simulink model "DigitalTwinUAV_R22"  (R2022a)
settings: Solver=VariableStepAuto  StartTime=0.0  StopTime=90  FixedStep=0.01  RelTol=1e-3
PreLoadFcn:
  | addpath(genpath('./images'));
InitFcn:
  | addpath(genpath('./model'));
  | QuadcopterParameters;
values from neighbouring files (symbols this model uses):
  m = 1.5    [QuadcopterParameters.m]    (also in QuadcopterParameters1.m; QuadcopterParameters_Gen.m = 1.2)
  trajColor = [0 0 0;              1 0 0;              0 0 1;]    [QuadcopterParameters.m]    (also in QuadcopterParameters1.m; QuadcopterParameters_Gen.m)
  xrot = 0    [QuadcopterParameters.m]    (also in QuadcopterParameters1.m; QuadcopterParameters_Gen.m)
  yrot = 0    [QuadcopterParameters.m]    (also in QuadcopterParameters1.m; QuadcopterParameters_Gen.m)
  zrot = 0    [QuadcopterParameters.m]    (also in QuadcopterParameters1.m; QuadcopterParameters_Gen.m)
undefined symbols (not defined in the file or in its folder): crane, excavator, uav, X, Y, Z
libraries: sm_lib x23, nesl_utility x1
(part 1 of 2)
settings Model: Creator=ADMIN  LastModifiedBy=ADMIN
settings SolverCC: MinimalZcImpactIntegration=on
settings SimscapeCC: SimscapeCompileComponentReuse=on
settings ExplorerConfigSet: InternalSimMechanicsExplorerSettings="<ExplorerConfiguration><canonicalview>default</canonicalview><AnimationSetting><BasePlaybackSpeed>1.0</BasePlaybackSpeed><PlaybackSpeedFactor>1.0</PlaybackSpeedFactor></AnimationSetting><TilePanel><TileInfo><Tiles Columns=\"1\" Count=\"1\" Rows=\"1\"><Column Weight=\"1\"/><Row Weight=\"1\"/><Tile Height=\"1\" Width=\"1\" X=\"0\" Y=\"0\"/></Tiles></TileInfo><SceneInfo><SceneViewer><BGColor><R>0.27843138575553894</R><G>0.756862759590148926</G><B>1</B></BGColor><Camera><DoPerspective>on</DoPerspective><Position><X>138.89503174773705</X><Y>141.338904454019598</Y><Z>58.1618377405307001</Z></Position><Center><X>60.3194201572761557</X><Y>73.694454858331909</Y><Z>-0.0339667202272622148</Z></Center><Up><X>-0.356422741563376222</X><Y>-0.336016505355418327</Y><Z>0.871811755727794013</Z></Up><ViewLimDist>1</ViewLimDist><YLim>0.466307658154998583</YLim><XLim>0.993847635057623302</XLim></Camera></SceneViewer></SceneInfo></TilePanel><MechEditorPanel><Cameras><Camera><Id>Camera1</Id><Value><Name>Camera</Name><NativeCamera><PositionKeyframeSet><Keyframe><Time>0</Time><Value><X>427.15819708198001</X><Y>-427.15819423097219</Y><Z>426.90819247014201</Z></Value></Keyframe><Keyframe><Time>0.79457934452222712</Time><Value><X>390.94235477737851</X><Y>-386.70665235425116</Y><Z>390.0308137752491</Z></Value></Keyframe><Keyframe><Time>2.7607911592394796</Time><Value><X>158.64332905928893</X><Y>-123.54772038663614</Y><Z>149.97829764303876</Z></Value></Keyframe><Keyframe><Time>5.5687271331598325</Time><Value><X>18.352849951551754</X><Y>24.396360824115767</Y><Z>18.562507619437909</Z></Value></Keyframe><Keyframe><Time>8.621944778587002</Time><Value><X>20.826011553668287</X><Y>30.414284305635885</Y><Z>22.10726949884149</Z></Value></Keyframe><Keyframe><Time>21.446938827871989</Time><Value><X>19.889419356045895</X><Y>44.10598770409257</Y><Z>15.738331202819449</Z></Value></Keyframe><Keyframe><Time>27.401526741577165</Time><Value><X>21.930325513031203</X><Y>49.554645689571032</Y><Z>15.972170552776927</Z></Value></Keyframe><Keyframe><Time>34.605538577791457</Time><Value><X>26.025912835327635</X><Y>57.985685802266083</Y><Z>15.892067554830771</Z></Value></Keyframe><Keyframe><Time>45.499317901054738</Time><Value><X>31.896560076715794</X><Y>65.244002145148229</Y><Z>15.465340540520041</Z></Value></Keyframe><Keyframe><Time>55.071901613661723</Time><Value><X>37.240526947587739</X><Y>68.058216295740905</Y><Z>16.878264808436938</Z></Value></Keyframe><Keyframe><Time>62.860219848906418</Time><Value><X>35.065406183068731</X><Y>62.163143721032611</Y><Z>16.14648566291422</Z></Value></Keyframe><Keyframe><Time>70.548436312612282</Time><Value><X>41.431101082419787</X><Y>65.763582084873633</Y><Z>15.666397795239471</Z></Value></Keyframe><Keyframe><Time>78.126717813603349</Time><Value><X>42.555026223671902</X><Y>67.92319371264098</Y><Z>16.748697346533454</Z></Value></Keyframe><Keyframe><Time>84.304620203487019</Time><Value><X>47.88954698511801</X><Y>72.641324967288227</Y><Z>16.299206866506246</Z></Value></Keyframe><Keyframe><Time>89.667208950866709</Time><Value><X>63.197259172121463</X><Y>84.566139055302173</Y><Z>18.486390887992304</Z></Value></Keyframe><Keyframe><Time>92.959131386818399</Time><Value><X>69.956308832017754</X><Y>89.839406171374179</Y><Z>19.43507026407455</Z></Value></Keyframe><Keyframe><Time>97.322347567853896</Time><Value><X>69.956308832017754</X><Y>89.839406171374179</Y><Z>19.43507026407455</Z></Value></Keyframe><Keyframe><Time>98.712529870538134</Time><Value><X>74.584383228853454</X><Y>87.281767315743537</Y><Z>18.165708290173569</Z></Value></Keyframe><Keyframe><Time>99.998699176458231</Time><Value><X>91.399732222435318</X><Y>137.62730154690249</Y><Z>39.166257857095417</Z></Value></Keyframe></PositionKeyframeSet><CenterKeyframeSet><Keyframe><Time>0</Time><Value><X>0.083335820948605033</X><Y>-0.083332969940784096</Y><Z>-0.16666879088938913</Z></Value></Keyframe><Keyframe><Time>0.79457934452222712</Time><Value><X>0.57379571983329924</X><Y>3.6619067032940507</Y><Z>-0.33774528229611178</Z></Value></Keyframe><Keyframe><Time>2.7607911592394796</Time><Value><X>8.66462376881978</X><Y>26.430984903833007</Y><Z>-0.00040764743039289897</Z></Value></Keyframe><Keyframe><Time>5.5687271331598325</Time><Value><X>-0.20970812157613494</X><Y>42.958918897243649</Y><Z>-5.0453689972584925e-05</Z></Value></Keyframe><Keyframe><Time>8.621944778587002</Time><Value><X>-1.2813180336776462</X><Y>52.521613892981804</Y><Z>-6.0088504437061374e-05</Z></Value></Keyframe><Keyframe><Time>21.446938827871989</Time><Value><X>4.1510453757688168</X><Y>59.844361684369609</Y><Z>-4.2777457625930992e-05</Z></Value></Keyframe><Keyframe><Time>27.401526741577165</Time><Value><X>5.958111547211292</X><Y>65.526859655390879</Y><Z>-4.3413042980944283e-05</Z></Value></Keyframe><Keyframe><Time>34.605538577791457</Time><Value><X>10.133802085177258</X><Y>73.877796552416413</Y><Z>-4.3195319602062909e-05</Z></Value></Keyframe><Keyframe><Time>45.499317901054738</Time><Value><X>31.445175359024709</X><Y>65.695386862839314</Y><Z>15.013955822828954</Z></Value></Keyframe><Keyframe><Time>55.071901613661723</Time><Value><X>57.580363961468976</X><Y>79.121527581700704</Y><Z>-4.337800287146365e-05</Z></Value></Keyframe><Keyframe><Time>62.860219848906418</Time><Value><X>56.144668811679956</X><Y>45.463359961310942</Y><Z>-6.1925334591705905e-05</Z></Value></Keyframe><Keyframe><Time>70.548436312612282</Time><Value><X>70.673607091545776</X><Y>33.834095876567901</Y><Z>-0.00016262240450970467</Z></Value></Keyframe><Keyframe><Time>78.126717813603349</Time><Value><X>73.053878820458976</X><Y>31.844243209726066</Y><Z>-0.00018157159788501076</Z></Value></Keyframe><Keyframe><Time>84.304620203487019</Time><Value><X>77.569891514658522</X><Y>37.530637514621176</Y><Z>-0.00017669869923864212</Z></Value></Keyframe><Keyframe><Time>89.667208950866709</Time><Value><X>96.860397210505056</X><Y>44.743962558486032</Y><Z>-0.00020040982668589891</Z></Value></Keyframe><Keyframe><Time>92.959131386818399</Time><Value><X>105.34696226184363</X><Y>47.97364649046682</Y><Z>-0.00021069440148835383</Z></Value></Keyframe><Keyframe><Time>97.322347567853896</Time><Value><X>105.34696226184349</X><Y>47.973646490466983</Y><Z>-0.00021069440141019413</Z></Value></Keyframe><Keyframe><Time>98.712529870538134</Time><Value><X>74.078241101652537</X><Y>85.981985203045838</Y><Z>17.6855975838644</Z></Value></Keyframe><Keyframe><Time>99.998699176458231</Time><Value><X>68.472813135391121</X><Y>78.75055976409854</Y><Z>17.418494284741232</Z></Value></Keyframe></CenterKeyframeSet><UpVectorKeyframeSet><Keyframe><Time>0</Time><Value><X>-0.40824829046386302</X><Y>0.40824829046386302</Y><Z>0.81649658092772603</Z></Value></Keyframe><Keyframe><Time>0.79457934452222712</Time><Value><X>-0.40824829046386302</X><Y>0.40824829046386302</Y><Z>0.81649658092772603</Z></Value></Keyframe><Keyframe><Time>2.7607911592394796</Time><Value><X>-0.40824829046386307</X><Y>0.40824829046386307</Y><Z>0.81649658092772615</Z></Value></Keyframe><Keyframe><Time>5.5687271331598325</Time><Value><X>-0.40824829046386302</X><Y>0.40824829046386302</Y><Z>0.81649658092772626</Z></Value></Keyframe><Keyframe><Time>8.621944778587002</Time><Value><X>-0.40824829046386302</X><Y>0.40824829046386302</Y><Z>0.81649658092772603</Z></Value></Keyframe><Keyframe><Time>21.446938827871989</Time><Value><X>-0.40824829046386329</X><Y>0.40824829046386335</Y><Z>0.81649658092772581</Z></Value></Keyframe><Keyframe><Time>27.401526741577165</Time><Value><X>-0.40824829046386346</X><Y>0.40824829046386346</Y><Z>0.81649658092772548</Z></Value></Keyframe><Keyframe><Time>34.605538577791457</Time><Value><X>-0.40824829046386324</X><Y>0.40824829046386335</Y><Z>0.81649658092772559</Z></Value></Keyframe><Keyframe><Time>45.499317901054738</Time><Value><X>-0.40824829046386291</X><Y>0.40824829046386307</Y><Z>0.81649658092772603</Z></Value></Keyframe><Keyframe><Time>55.071901613661723</Time><Value><X>0.54474303700342208</X><Y>0.22917420964799837</Y><Z>0.80668098110002795</Z></Value></Keyframe><Keyframe><Time>62.860219848906418</Time><Value><X>0.33216731732567528</X><Y>-0.40455279321782145</Y><Z>0.85205745745244355</Z></Value></Keyframe><Keyframe><Time>70.548436312612282</Time><Value><X>0.22596689908931417</X><Y>-0.2544284640580029</Y><Z>0.94032181575939477</Z></Value></Keyframe><Keyframe><Time>78.126717813603349</Time><Value><X>0.24849257206902248</X><Y>-0.22707675815979272</Y><Z>0.94164090158093749</Z></Value></Keyframe><Keyframe><Time>84.304620203487019</Time><Value><X>0.24849257206902248</X><Y>-0.22707675815979275</Y><Z>0.94164090158093749</Z></Value></Keyframe><Keyframe><Time>89.667208950866709</Time><Value><X>0.24849257206902245</X><Y>-0.22707675815979272</Y><Z>0.94164090158093749</Z></Value></Keyframe><Keyframe><Time>92.959131386818399</Time><Value><X>0.24849257206902245</X><Y>-0.22707675815979272</Y><Z>0.94164090158093749</Z></Value></Keyframe><Keyframe><Time>97.322347567853896</Time><Value><X>0.24849257206902245</X><Y>-0.2270767581597927</Y><Z>0.94164090158093749</Z></Value></Keyframe><Keyframe><Time>98.712529870538134</Time><Value><X>-0.11527700489361359</X><Y>-0.30437604885319575</Y><Z>0.945550862210635</Z></Value></Keyframe><Keyframe><Time>99.998699176458231</Time><Value><X>-0.11527700489361427</X><Y>-0.30437604885319752</Y><Z>0.94555086221063411</Z></Value></Keyframe></UpVectorKeyframeSet></NativeCamera></Value></Camera><Camera><Id>Camera2</Id><Value><Name>Camera2</Name><NativeCamera><PositionKeyframeSet><Keyframe><Time>0</Time><Value><X>229.42211701613911</X><Y>-181.57056116872968</Y><Z>204.32036374857904</Z></Value></Keyframe><Keyframe><Time>1.000273018622585</Time><Value><X>197.55127895537666</X><Y>-148.90451616468175</Y><Z>172.77519677524185</Z></Value></Keyframe><Keyframe><Time>1.9998413608981176</Time><Value><X>152.00964089221299</X><Y>-103.76251203481223</Y><Z>129.85617953038943</Z></Value></Keyframe><Keyframe><Time>2.9997698665509209</Time><Value><X>91.305579739639839</X><Y>-43.282088723920879</Y><Z>76.593292484691659</Z></Value></Keyframe><Keyframe><Time>4.0000437696161804</Time><Value><X>63.675921698844178</X><Y>-16.182993482292915</Y><Z>53.58702589586548</Z></Value></Keyframe><Keyframe><Time>5.0001784288957127</Time><Value><X>30.124862570999188</X><Y>14.013191865709302</Y><Z>25.811716641985729</Z></Value></Keyframe><Keyframe><Time>6.0001514418482849</Time><Value><X>23.245853605889877</X><Y>21.271258776668272</Y><Z>19.318526585402044</Z></Value></Keyframe><Keyframe><Time>7.0000336661717562</Time><Value><X>26.868198636186534</X><Y>25.847341414168035</Y><Z>20.272264192605149</Z></Value></Keyframe><Keyframe><Time>8.000135993662056</Time><Value><X>26.868198636186534</X><Y>25.847341414168035</Y><Z>20.272264192605149</Z></Value></Keyframe><Keyframe><Time>12.000060521855515</Time><Value><X>26.327006126208872</X><Y>27.710686973014656</Y><Z>22.676802261429437</Z></Value></Keyframe><Keyframe><Time>14.999735667122877</Time><Value><X>28.295728944359858</X><Y>27.480602511595009</Y><Z>20.477994981858799</Z></Value></Keyframe><Keyframe><Time>16.000205697859094</Time><Value><X>30.310341141247953</X><Y>29.879687394354729</Y><Z>20.862467667730424</Z></Value></Keyframe><Keyframe><Time>18</Time><Value><X>26.770305336655007</X><Y>35.477008620321833</Y><Z>18.099995586746186</Z></Value></Keyframe><Keyframe><Time>20.00000304433263</Time><Value><X>27.472962547810489</X><Y>37.810046819920885</Y><Z>19.730376575189759</Z></Value></Keyframe><Keyframe><Time>22.000224197946089</Time><Value><X>26.9792421697192</X><Y>37.813168521453861</Y><Z>19.792629719475226</Z></Value></Keyframe><Keyframe><Time>24.00016511781271</Time><Value><X>24.889252072130148</X><Y>35.375391905924594</Y><Z>19.531772772823498</Z></Value></Keyframe><Keyframe><Time>26.000093825701278</Time><Value><X>23.428642671004315</X><Y>37.197471869241348</Y><Z>17.738764614919702</Z></Value></Keyframe><Keyframe><Time>27.999962847707238</Time><Value><X>20.387005350891794</X><Y>42.79597426548974</Y><Z>16.352519575890927</Z></Value></Keyframe><Keyframe><Time>29.999690502428876</Time><Value><X>19.277686757978806</X><Y>43.962422440853544</Y><Z>16.146129384446127</Z></Value></Keyframe><Keyframe><Time>31.999734624362802</Time><Value><X>19.72713372758853</X><Y>48.573829120962806</Y><Z>18.193453440233878</Z></Value></Keyframe><Keyframe><Time>33.999673255119724</Time><Value><X>19.782458532238007</X><Y>52.112301987038968</Y><Z>19.642549513946232</Z></Value></Keyframe><Keyframe><Time>36</Time><Value><X>21.55325105949694</X><Y>53.949829712966483</Y><Z>19.171654687490552</Z></Value></Keyframe><Keyframe><Time>37.99983496478324</Time><Value><X>23.437474942885132</X><Y>55.627893150481249</Y><Z>16.994152381120042</Z></Value></Keyframe><Keyframe><Time>39.999704023181188</Time><Value><X>24.998911581156065</X><Y>62.488557443752292</Y><Z>18.940639854790781</Z></Value></Keyframe><Keyframe><Time>42.000166465258886</Time><Value><X>28.409434539739252</X><Y>69.214963954081696</Y><Z>20.058059863527468</Z></Value></Keyframe><Keyframe><Time>43.999717964839682</Time><Value><X>34.699289096189688</X><Y>70.961283734018451</Y><Z>18.466447327852634</Z></Value></Keyframe><Keyframe><Time>45.999916464499805</Time><Value><X>36.40543007932564</X><Y>71.857960605414263</Y><Z>17.64562444618441</Z></Value></Keyframe><Keyframe><Time>48.000128581837849</Time><Value><X>39.43057749066287</X><Y>72.257422850905826</Y><Z>18.739347841870078</Z></Value></Keyframe><Keyframe><Time>49.99992478618293</Time><Value><X>43.422403550355781</X><Y>73.212796107446692</Y><Z>16.439241194456741</Z></Value></Keyframe><Keyframe><Time>51.999674329862636</Time><Value><X>46.934269420811198</X><Y>73.396555233271229</Y><Z>16.005507762443312</Z></Value></Keyframe><Keyframe><Time>54</Time><Value><X>49.102122803066699</X><Y>78.463229181998017</Y><Z>17.60108062581412</Z></Value></Keyframe><Keyframe><Time>56.000405512171703</Time><Value><X>50.933014881578096</X><Y>78.223728424998271</Y><Z>17.735828542058144</Z></Value></Keyframe><Keyframe><Time>57.999833678854806</Time><Value><X>53.835348032966493</X><Y>76.818838883930439</Y><Z>16.905995306639007</Z></Value></Keyframe><Keyframe><Time>59.99979126155737</Time><Value><X>61.626438596615735</X><Y>77.152448025005825</Y><Z>20.076073882268343</Z></Value></Keyframe><Keyframe><Time>61.999963873580292</Time><Value><X>61.969626521341368</X><Y>78.283733041699435</Y><Z>18.229640876326858</Z></Value></Keyframe><Keyframe><Time>65.999733038800883</Time><Value><X>69.166882183227898</X><Y>88.998353875388489</Y><Z>24.848351588577749</Z></Value></Keyframe><Keyframe><Time>70.000024012162029</Time><Value><X>72.56719371536758</X><Y>87.651305544240998</Y><Z>21.960175902186091</Z></Value></Keyframe><Keyframe><Time>75.000250424912963</Time><Value><X>80.058475334563909</X><Y>92.123433446463935</Y><Z>23.018878398528422</Z></Value></Keyframe><Keyframe><Time>80.000129153530565</Time><Value><X>81.377418765025041</X><Y>91.152346896609615</Y><Z>22.449006776150824</Z></Value></Keyframe><Keyframe><Time>85.00016728403746</Time><Value><X>83.985608228435296</X><Y>87.819241830809133</Y><Z>23.05563029704135</Z></Value></Keyframe><Keyframe><Time>86.000313905552019</Time><Value><X>94.607344859457129</X><Y>98.816411737799271</Y><Z>29.324817264882864</Z></Value></Keyframe><Keyframe><Time>87.000040311365154</Time><Value><X>107.47852215936517</X><Y>110.35675145021976</Y><Z>36.94655917351227</Z></Value></Keyframe><Keyframe><Time>88.000098835330618</Time><Value><X>117.80884802291686</X><Y>118.56459591723726</Y><Z>41.509985959976191</Z></Value></Keyframe><Keyframe><Time>89.000164588923155</Time><Value><X>138.89503174773705</X><Y>141.3389044540196</Y><Z>58.1618377405307</Z></Value></Keyframe><Keyframe><Time>90</Time><Value><X>138.89503174773705</X><Y>141.3389044540196</Y><Z>58.1618377405307</Z></Value></Keyframe></PositionKeyframeSet><CenterKeyframeSet><Keyframe><Time>0</Time><Value><X>31.551215256709213</X><Y>16.300340590700216</Y><Z>6.4494619891492846</Z></Value></Keyframe><Keyframe><Time>1.000273018622585</Time><Value><X>31.225629910397572</X><Y>17.421132880297336</Y><Z>6.449547730262907</Z></Value></Keyframe><Keyframe><Time>1.9998413608981176</Time><Value><X>28.603125747811816</X><Y>19.644003109588937</Y><Z>6.4496643859883562</Z></Value></Keyframe><Keyframe><Time>2.9997698665509209</Time><Value><X>21.162096411742439</X><Y>26.861394603976521</Y><Z>6.4498091567943305</Z></Value></Keyframe><Keyframe><Time>4.0000437696161804</Time><Value><X>10.097994763739074</X><Y>37.39493345281219</Y><Z>0.0090989607604328171</Z></Value></Keyframe><Keyframe><Time>5.0001784288957127</Time><Value><X>4.2543460249819205</X><Y>39.883708411726559</Y><Z>-0.05879990403151325</Z></Value></Keyframe><Keyframe><Time>6.0001514418482849</Time><Value><X>3.8660014095456816</X><Y>40.651110973012464</Y><Z>-0.061325610942130737</Z></Value></Keyframe><Keyframe><Time>7.0000336661717562</Time><Value><X>8.6220160008767692</X><Y>44.0935240494778</Y><Z>2.0260815572954023</Z></Value></Keyframe><Keyframe><Time>8.000135993662056</Time><Value><X>8.6220160008767692</X><Y>44.0935240494778</Y><Z>2.0260815572954023</Z></Value></Keyframe><Keyframe><Time>12.000060521855515</Time><Value><X>3.6196002136333156</X><Y>50.418092885590212</Y><Z>-0.03060365114610164</Z></Value></Keyframe><Keyframe><Time>14.999735667122877</Time><Value><X>9.8435740796902387</X><Y>45.932757376264625</Y><Z>2.025840117189194</Z></Value></Keyframe><Keyframe><Time>16.000205697859094</Time><Value><X>9.3757361975952556</X><Y>50.814292338007419</Y><Z>-0.072137275922251831</Z></Value></Keyframe><Keyframe><Time>18</Time><Value><X>8.5950745814058997</X><Y>53.652239375570929</Y><Z>-0.075235168502903349</Z></Value></Keyframe><Keyframe><Time>20.00000304433263</Time><Value><X>7.6933622646033051</X><Y>57.589647103128058</Y><Z>-0.049223708017400725</Z></Value></Keyframe><Keyframe><Time>22.000224197946089</Time><Value><X>7.782901084608234</X><Y>63.428094772265339</Y><Z>-0.038654727826529012</Z></Value></Keyframe><Keyframe><Time>24.00016511781271</Time><Value><X>13.913441370701982</X><Y>66.048311344047619</Y><Z>-0.092996799423143983</Z></Value></Keyframe><Keyframe><Time>26.000093825701278</Time><Value><X>23.072997760502972</X><Y>76.610494481889674</Y><Z>-0.14044226985273767</Z></Value></Keyframe><Keyframe><Time>27.999962847707238</Time><Value><X>46.056529688525444</X><Y>98.918869182276225</Y><Z>-0.14817845045401867</Z></Value></Keyframe><Keyframe><Time>29.999690502428876</Time><Value><X>38.716876529679176</X><Y>72.170423114431159</Y><Z>2.6247209653232257</Z></Value></Keyframe><Keyframe><Time>31.999734624362802</Time><Value><X>45.151887248357326</X><Y>74.962821820866424</Y><Z>-0.14866172727078464</Z></Value></Keyframe><Keyframe><Time>33.999673255119724</Time><Value><X>43.931163511354093</X><Y>67.582519550125397</Y><Z>-0.12866311492846805</Z></Value></Keyframe><Keyframe><Time>36</Time><Value><X>43.067358977399621</X><Y>65.689847250674404</Y><Z>-0.14765266506854857</Z></Value></Keyframe><Keyframe><Time>37.99983496478324</Time><Value><X>49.609993385732579</X><Y>60.617525110879157</Y><Z>-0.17407851231168436</Z></Value></Keyframe><Keyframe><Time>39.999704023181188</Time><Value><X>51.174089651313913</X><Y>54.359329955310301</Y><Z>-0.13671416647383694</Z></Value></Keyframe><Keyframe><Time>42.000166465258886</Time><Value><X>50.696412624780663</X><Y>51.690721304467345</Y><Z>-0.19360313930595296</Z></Value></Keyframe><Keyframe><Time>43.999717964839682</Time><Value><X>48.011280497921405</X><Y>51.102412583964153</Y><Z>-0.16139757887929562</Z></Value></Keyframe><Keyframe><Time>45.999916464499805</Time><Value><X>42.027850149919999</X><Y>46.970089378998651</Y><Z>-0.15914948743381885</Z></Value></Keyframe><Keyframe><Time>48.000128581837849</Time><Value><X>39.876142820446589</X><Y>48.019983028776402</Y><Z>0.23639313961458086</Z></Value></Keyframe><Keyframe><Time>49.99992478618293</Time><Value><X>43.155499075415847</X><Y>39.116884003467959</Y><Z>-0.16719766176567674</Z></Value></Keyframe><Keyframe><Time>51.999674329862636</Time><Value><X>46.674274865613164</X><Y>40.183356003321087</Y><Z>-0.17100514472535622</Z></Value></Keyframe><Keyframe><Time>54</Time><Value><X>40.19857623926984</X><Y>40.436259613424383</Y><Z>-0.17876690208317214</Z></Value></Keyframe><Keyframe><Time>56.000405512171703</Time><Value><X>30.565909477925825</X><Y>46.68510342886735</Y><Z>-0.10370858691696228</Z></Value></Keyframe><Keyframe><Time>57.999833678854806</Time><Value><X>34.360890580665838</X><Y>46.662486352800599</Y><Z>-0.1516719416811334</Z></Value></Keyframe><Keyframe><Time>59.99979126155737</Time><Value><X>34.620682256769918</X><Y>52.339801741754989</Y><Z>-0.14573991684069298</Z></Value></Keyframe><Keyframe><Time>61.999963873580292</Time><Value><X>37.429707408008767</X><Y>55.736675847070806</Y><Z>-0.14576282317352351</Z></Value></Keyframe><Keyframe><Time>65.999733038800883</Time><Value><X>35.747406970283912</X><Y>58.292840317630379</Y><Z>-0.17603197304744356</Z></Value></Keyframe><Keyframe><Time>70.000024012162029</Time><Value><X>42.962834940698002</X><Y>60.451086691843429</Y><Z>-0.20746210986618863</Z></Value></Keyframe><Keyframe><Time>75.000250424912963</Time><Value><X>49.082196705445583</X><Y>63.662706958248734</Y><Z>-0.17604829579010328</Z></Value></Keyframe><Keyframe><Time>80.000129153530565</Time><Value><X>51.181542102007761</X><Y>63.408646723078604</Y><Z>-0.16155771596307034</Z></Value></Keyframe><Keyframe><Time>85.00016728403746</Time><Value><X>52.961369683396633</X><Y>59.314450202757428</Y><Z>-0.17520861085703388</Z></Value></Keyframe><Keyframe><Time>86.000313905552019</Time><Value><X>55.165568234182842</X><Y>62.577661751672807</Y><Z>-0.20904406399046849</Z></Value></Keyframe><Keyframe><Time>87.000040311365154</Time><Value><X>58.034445661262353</X><Y>64.927978209780093</Y><Z>-0.076988540954268103</Z></Value></Keyframe><Keyframe><Time>88.000098835330618</Time><Value><X>62.185868062220734</X><Y>67.458701691688489</Y><Z>-0.14030257710807348</Z></Value></Keyframe><Keyframe><Time>89.000164588923155</Time><Value><X>60.319420157276156</X><Y>73.694454858331909</Y><Z>-0.033966720227262215</Z></Value></Keyframe><Keyframe><Time>90</Time><Value><X>60.319420157276156</X><Y>73.694454858331909</Y><Z>-0.033966720227262215</Z></Value></Keyframe></CenterKeyframeSet><UpVectorKeyframeSet><Keyframe><Time>0</Time><Value><X>-0.40824829046386285</X><Y>0.40824829046386285</Y><Z>0.81649658092772637</Z></Value></Keyframe><Keyframe><Time>1.000273018622585</Time><Value><X>-0.40824829046386285</X><Y>0.40824829046386285</Y><Z>0.81649658092772637</Z></Value></Keyframe><Keyframe><Time>1.9998413608981176</Time><Value><X>-0.4082482904638628</X><Y>0.4082482904638628</Y><Z>0.81649658092772615</Z></Value></Keyframe><Keyframe><Time>2.9997698665509209</Time><Value><X>-0.4082482904638628</X><Y>0.4082482904638628</Y><Z>0.81649658092772637</Z></Value></Keyframe><Keyframe><Time>4.0000437696161804</Time><Value><X>-0.4082482904638628</X><Y>0.4082482904638628</Y><Z>0.81649658092772637</Z></Value></Keyframe><Keyframe><Time>5.0001784288957127</Time><Value><X>-0.4082482904638628</X><Y>0.40824829046386285</Y><Z>0.81649658092772626</Z></Value></Keyframe><Keyframe><Time>6.0001514418482849</Time><Value><X>-0.40824829046386274</X><Y>0.4082482904638628</Y><Z>0.81649658092772626</Z></Value></Keyframe><Keyframe><Time>7.0000336661717562</Time><Value><X>-0.4082482904638628</X><Y>0.4082482904638628</Y><Z>0.81649658092772637</Z></Value></Keyframe><Keyframe><Time>8.000135993662056</Time><Value><X>-0.4082482904638628</X><Y>0.4082482904638628</Y><Z>0.81649658092772637</Z></Value></Keyframe><Keyframe><Time>12.000060521855515</Time><Value><X>-0.40824829046386285</X><Y>0.4082482904638628</Y><Z>0.81649658092772626</Z></Value></Keyframe><Keyframe><Time>14.999735667122877</Time><Value><X>-0.40824829046386285</X><Y>0.4082482904638628</Y><Z>0.81649658092772626</Z></Value></Keyframe><Keyframe><Time>16.000205697859094</Time><Value><X>-0.40824829046386285</X><Y>0.40824829046386274</Y><Z>0.81649658092772648</Z></Value></Keyframe><Keyframe><Time>18</Time><Value><X>-0.40824829046386291</X><Y>0.4082482904638628</Y><Z>0.81649658092772626</Z></Value></Keyframe><Keyframe><Time>20.00000304433263</Time><Value><X>-0.40824829046386285</X><Y>0.40824829046386274</Y><Z>0.81649658092772626</Z></Value></Keyframe><Keyframe><Time>22.000224197946089</Time><Value><X>-0.2076415760691887</X><Y>0.49678828253428997</Y><Z>0.8426662318048197</Z></Value></Keyframe><Keyframe><Time>24.00016511781271</Time><Value><X>-0.10349153115718084</X><Y>0.5095047257952674</Y><Z>0.85422153881240426</Z></Value></Keyframe><Keyframe><Time>26.000093825701278</Time><Value><X>0.01724342445728275</X><Y>0.41318482538090323</Y><Z>0.91048391769868098</Z></Value></Keyframe><Keyframe><Time>27.999962847707238</Time><Value><X>0.067872605599444649</X><Y>0.25272182893157097</Y><Z>0.96515542095075224</Z></Value></Keyframe><Keyframe><Time>29.999690502428876</Time><Value><X>0.1909138696933684</X><Y>0.31420726264793852</Y><Z>0.92996004777516816</Z></Value></Keyframe><Keyframe><Time>31.999734624362802</Time><Value><X>0.25943152749458853</X><Y>0.37007666749622292</Y><Z>0.89204178305543236</Z></Value></Keyframe><Keyframe><Time>33.999673255119724</Time><Value><X>0.46197420427831631</X><Y>0.33062684214562105</Y><Z>0.82296155793222292</Z></Value></Keyframe><Keyframe><Time>36</Time><Value><X>0.60437195743408978</X><Y>0.17243437041644957</Y><Z>0.77781805389587721</Z></Value></Keyframe><Keyframe><Time>37.99983496478324</Time><Value><X>0.53647232249382293</X><Y>0.07747352789652838</Y><Z>0.8403542703368323</Z></Value></Keyframe><Keyframe><Time>39.999704023181188</Time><Value><X>0.53033272477981597</X><Y>-0.21618020577307623</Y><Z>0.81976418539695095</Z></Value></Keyframe><Keyframe><Time>42.000166465258886</Time><Value><X>0.45656040875993176</X><Y>-0.35972693068730127</Y><Z>0.81372546260471512</Z></Value></Keyframe><Keyframe><Time>43.999717964839682</Time><Value><X>0.23350554221511466</X><Y>-0.57736166807542344</Y><Z>0.78238651956177641</Z></Value></Keyframe><Keyframe><Time>45.999916464499805</Time><Value><X>0.12374729915826878</X><Y>-0.5587224608187823</Y><Z>0.82007061752487997</Z></Value></Keyframe><Keyframe><Time>48.000128581837849</Time><Value><X>-0.033736250392236287</X><Y>-0.60684320495640887</Y><Z>0.79410527640087269</Z></Value></Keyframe><Keyframe><Time>49.99992478618293</Time><Value><X>0.0013892956227967378</X><Y>-0.43788423502487994</Y><Z>0.89903029235635246</Z></Value></Keyframe><Keyframe><Time>51.999674329862636</Time><Value><X>0.0013892956227967387</X><Y>-0.43788423502487972</Y><Z>0.89903029235635223</Z></Value></Keyframe><Keyframe><Time>54</Time><Value><X>-0.085296391303142496</X><Y>-0.40554749780702559</Y><Z>0.91008557435722603</Z></Value></Keyframe><Keyframe><Time>56.000405512171703</Time><Value><X>-0.19674286973940341</X><Y>-0.38337748613608125</Y><Z>0.90239345428182427</Z></Value></Keyframe><Keyframe><Time>57.999833678854806</Time><Value><X>-0.19674286973940347</X><Y>-0.38337748613608141</Y><Z>0.90239345428182438</Z></Value></Keyframe><Keyframe><Time>59.99979126155737</Time><Value><X>-0.36489842484907264</X><Y>-0.31645882291525435</Y><Z>0.87561575644900147</Z></Value></Keyframe><Keyframe><Time>61.999963873580292</Time><Value><X>-0.36489842484907264</X><Y>-0.31645882291525435</Y><Z>0.87561575644900158</Z></Value></Keyframe><Keyframe><Time>65.999733038800883</Time><Value><X>-0.3648984248490727</X><Y>-0.31645882291525446</Y><Z>0.87561575644900169</Z></Value></Keyframe><Keyframe><Time>70.000024012162029</Time><Value><X>-0.36489842484907259</X><Y>-0.3164588229152544</Y><Z>0.87561575644900147</Z></Value></Keyframe><Keyframe><Time>75.000250424912963</Time><Value><X>-0.3648984248490727</X><Y>-0.31645882291525446</Y><Z>0.87561575644900169</Z></Value></Keyframe><Keyframe><Time>80.000129153530565</Time><Value><X>-0.3648984248490727</X><Y>-0.31645882291525446</Y><Z>0.87561575644900169</Z></Value></Keyframe><Keyframe><Time>85.00016728403746</Time><Value><X>-0.36489842484907276</X><Y>-0.31645882291525457</Y><Z>0.87561575644900158</Z></Value></Keyframe><Keyframe><Time>86.000313905552019</Time><Value><X>-0.3648984248490727</X><Y>-0.31645882291525451</Y><Z>0.87561575644900158</Z></Value></Keyframe><Keyframe><Time>87.000040311365154</Time><Value><X>-0.36489842484907276</X><Y>-0.31645882291525457</Y><Z>0.87561575644900169</Z></Value></Keyframe><Keyframe><Time>88.000098835330618</Time><Value><X>-0.36489842484907264</X><Y>-0.31645882291525446</Y><Z>0.87561575644900147</Z></Value></Keyframe><Keyframe><Time>89.000164588923155</Time><Value><X>-0.35642274156337622</X><Y>-0.33601650535541833</Y><Z>0.87181175572779401</Z></Value></Keyframe><Keyframe><Time>90</Time><Value><X>-0.35642274156337622</X><Y>-0.33601650535541833</Y><Z>0.87181175572779401</Z></Value></Keyframe></UpVectorKeyframeSet></NativeCamera></Value></Camera></Cameras><GfxPanelCameraMap><MapElement CameraMLId=\"Camera2\" GfxPanelIndex=\"0\"/></GfxPanelCameraMap><VideoCreator><PlaybackSpeedRatio>1.0</PlaybackSpeedRatio><FrameRate>60</FrameRate><VideoFormat>MPEG-4</VideoFormat><FrameSize>[1920 1080]</FrameSize></VideoCreator></MechEditorPanel></ExplorerConfiguration>"

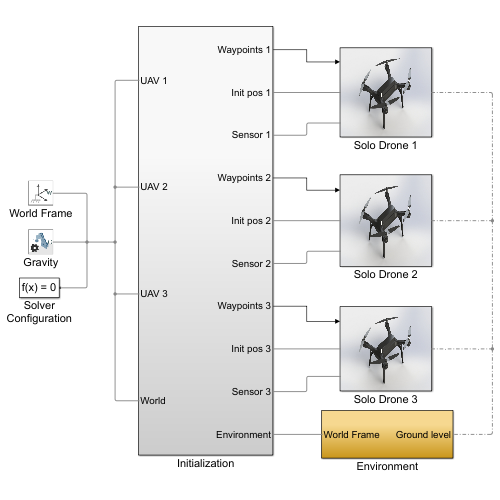
[thumbnail: Simulink's stored preview of the top-level diagram]
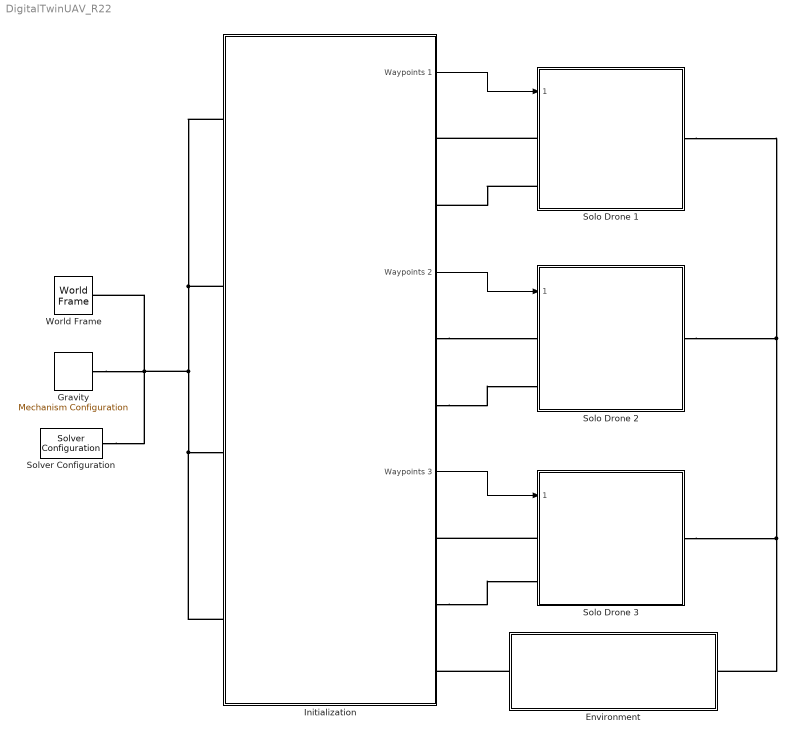
== system DigitalTwinUAV_R22 ==
  Environment : Subsystem
  Gravity : sm_lib/Utilities/Mechanism Configuration  UniformGravity=Constant  GravityVector=[0 0 -9.80665]  GravityUnits=m/s^2  LinearizationDelta=0.001  JointModeTransitionNonlinearIterations=2
  Initialization : Subsystem
      settings: PortSchema="{\"entries\":[{\"content\":{\"sides\":[{\"content\":{\"connectorIds\":[\"LConn1\",\"LConn2\",\"LConn3\",\"LConn4\"]},\"type\":\"ConnectorPlacement.EquallySpacedRectSide\",\"uuid\":\"5d0b77d9-9baf-460c-acbb-ff0e865e14b9\"},{\"content\":{\"connectorIds\":[\"Out1\",\"RConn1\",\"RConn2\",\"Out2\",\"RConn3\",\"RConn4\",\"Out3\",\"RConn5\",\"RConn6\",\"RConn7\"],\"side\":\"RIGHT\"},\"type\":\"ConnectorPlacement.EquallySpacedRectSide\",\"uuid\":\"e00fcb6a-2700-42c1-8e7b-fc55a4f923c3\"},{\"content\":{\"connectorIds\":[],\"side\":\"TOP\"},\"type\":\"ConnectorPlacement.EquallySpacedRectSide\",\"uuid\":\"a46608a6-d63a-4a87-980e-43f69080d525\"}]},\"type\":\"ConnectorPlacement.EquallySpacedConnector\",\"uuid\":\"0f1923d5-db6f-44c1-a252-23e77ab8a03f\"}],\"packageUris\":[\"http://schema.mathworks.com/mf0/Connector/R2020b\"],\"version\":\"1.0\"}"
  Solo Drone 1 : Subsystem  ReferencedSubsystem=UAV_R22a
  Solo Drone 2 : Subsystem  ReferencedSubsystem=UAV_R22a
  Solo Drone 3 : Subsystem  ReferencedSubsystem=UAV_R22a
  Solver Configuration : nesl_utility/Solver Configuration  PhysicalDomain=network_engine_domain  SubClassName=solver  LeftPortType=input  RightPortType=generic  Tones=[]  Harmonics=[]  SimulateNoise=off  Profile=off  UseLocalSampling=off  EnableSwitchedLinearOptims=on  FrequencyDomain=off  UseCCode=off  RelTol=0.001  AbsTol=1e-06  MinStep=1e-09  ToWorkspace=off  RevertToSquareIcSolve=off  NumHomotopyIterations=100  PhasorMode=off  PhasorModeNumHarmonics=1  IndexReductionMethod=DerivativeReplacement  DoDC=off  ResidualTolerance=1e-09  UseLocalSolver=off  LocalSolverChoice=NE_BACKWARD_EULER_ADVANCER  LocalSolverSampleTime=Ts  DoFixedCost=off  MaxNonlinIter=3  MaxModeIter=2  ComputeImpulses=off  ImpulseIterations=2  LinearAlgebra=auto  LinearAlgebraNumThread=0  EquationFormulation=NE_TIME_EF  DelaysMemoryBudget=1024  AutomaticFiltering=on  FilteringTimeConstant=0.001  PartitionStorageMethod=AS_NEEDED  PartitionMemoryBudget=1024  PartitionMethod=ROBUST
      settings: SourceProductBaseCode=SS,PW,VE
  World Frame : sm_lib/Frames and Transforms/World Frame
  wires:
  Initialization/1(Waypoints 1) -> Solo Drone 1/1
  Initialization/2(Waypoints 2) -> Solo Drone 2/1
  Initialization/3(Waypoints 3) -> Solo Drone 3/1
  connections:
  Solo Drone 1/RConn1 -- Solo Drone 2/RConn1 -- Solo Drone 3/RConn1 -- Environment/LConn1
  Solver Configuration/RConn1 -- Initialization/LConn3 -- Initialization/LConn4 -- Initialization/LConn2 -- Initialization/LConn1 -- Gravity/RConn1 -- World Frame/RConn1
  Solo Drone 1/LConn1 -- Initialization/RConn1
  Initialization/RConn3 -- Solo Drone 2/LConn1
  Solo Drone 3/LConn1 -- Initialization/RConn5
  Environment/RConn1 -- Initialization/RConn7
  Solo Drone 1/LConn2 -- Initialization/RConn2
  Initialization/RConn4 -- Solo Drone 2/LConn2
  Initialization/RConn6 -- Solo Drone 3/LConn2

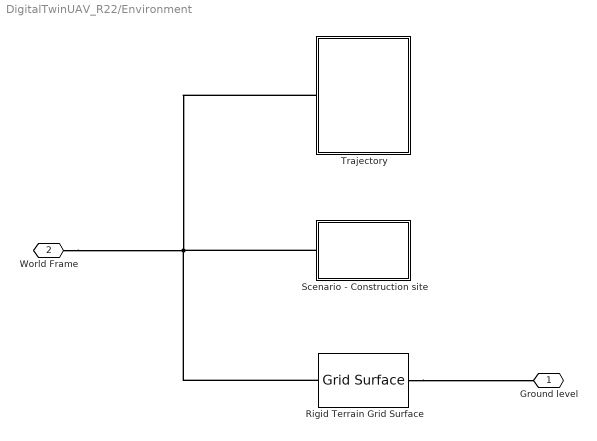
== system DigitalTwinUAV_R22/Environment ==
  Rigid Terrain Grid Surface : sm_lib/Curves and Surfaces/Grid Surface  XGridVector=xg  XGridVectorUnits=m  YGridVector=yg  YGridVectorUnits=m  ZHeights=z_heights  ZHeightsUnits=m  GraphicType=FromGeometry  GraphicVisPropType=SimpleVisualProperties  GraphicDiffuseColor=[0.9294 0.6941 0.1255]  GraphicOpacity=1.0  GraphicSpecularColor=[0.5 0.5 0.5 1.0]  GraphicAmbientColor=[0.15 0.15 0.15 1.0]  GraphicEmissiveColor=[0.0 0.0 0.0 1.0]  GraphicShininess=75
      settings: SourceProductBaseCode=MS
  Scenario - Construction site : Subsystem
  Trajectory : Subsystem
  Ground level : PMIOPort  Side=Left
  World Frame : PMIOPort  Port=2  Side=Right
  connections:
  Rigid Terrain Grid Surface/RConn1 -- Ground level/RConn1
  Rigid Terrain Grid Surface/LConn1 -- World Frame/RConn1 -- Trajectory/LConn1 -- Scenario - Construction site/LConn1
